simulink model "akku_schaetzung"  (R2021a)
settings: Solver=VariableStepAuto  StartTime=0.0  StopTime=time_est  RelTol=1e-3
values from neighbouring files (symbols this model uses):
  a = param    [temp.m]    (also in toolbox_ident.m = phi'*phi\phi'*u_oc)
  current = main_data{cur_ind}.Values    [check_output.m]    (also in init.m; init_2.m; init_3.m; power_energy.m)
  Delta = 8e-3    (= 0.008)    [check_output.m]    (also in init.m = volt_clean.Time(2)-volt_clean.Time(1); init_2.m; temp.m; toolbox_ident.m)
  P0 = eye(5); P0(1,1)=(0.03*x0(1))^2;P0(2,2)=(0.03*x0(2))^2;P0(3,3)=(0.03*x0(3))^2    [check_output.m]    (also in init.m; init_2.m; init_3.m = eye(6); P0(1,1)=(0.03*x0(1))^2;P0(2,2)=(0.03*x0(2))^2;P0(3,3; temp.m)
  Q_e = 2.9*3600    (= 10440)    [check_output.m]    (also in init_2.m; temp.m; toolbox_ident.m)
  voltage = main_data{volt_ind}.Values    [check_output.m]    (also in init.m; init_2.m; init_3.m; power_energy.m)
  W_k = 0.0*eye(5)    [check_output.m]    (also in init.m = 0.0*eye(6); init_2.m; init_3.m = 0.0*eye(6); temp.m)
  x0 = [1/param_conv(1); 1/param_conv(2); 1/param_conv(3); soc_0; 0]    [check_output.m]    (also in init.m = [1/790.27; 1/0.0126; 1/0.0086; 1/(2.9*3600); 0.5; 0]; init_2.m = [2/790.27; 1/0.0126/2; 1/0.0086/2; 0.5; 0]; init_3.m = [2/790.27; 1/2/0.0126; 1/2/0.0086; 1/(2.9*3600); 0.5; 0]; temp.m = [2/790.27; 1/0.0126/2; 1/0.0086/2; 0.5; 0])
  Z_k = var(static_volt)    [check_output.m]    (also in init.m = 0.02; init_2.m; init_3.m; temp.m)
undefined symbols (not defined in the file or in its folder): ind_val
libraries: simulink x2
settings Model: Creator=saleh  LastModifiedBy=saleh
settings SolverCC: AlgebraicLoopSolver=TrustRegion
settings DebuggingCC: SFMachineParentedDataDiag=warning

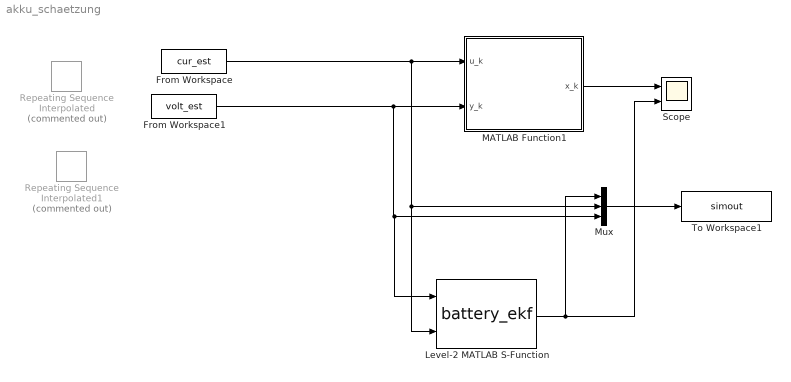
== system akku_schaetzung ==
  From Workspace : FromWorkspace  VariableName=cur_est  SampleTime=Delta
  From Workspace1 : FromWorkspace  VariableName=volt_est  SampleTime=Delta
  Level-2 MATLAB S-Function : M-S-Function  FunctionName=battery_ekf  Parameters=Delta, x0, P0, a, Z_k, W_k, Q_e
  MATLAB Function1 : MATLAB Function  TreatAsAtomicUnit=on
  Mux : Mux  Inputs=3
  Repeating Sequence Interpolated : simulink/Sources/Repeating Sequence Interpolated  Commented=on  OutValues=current.Data(1:ind_val)  TimeValues=current.Time(1:ind_val)  LookUpMeth=Interpolation-Use End Values  tsamp=Delta  OutMin=[]  OutMax=[]  OutDataTypeStr=double  OutputDataTypeScalingMode=double  OutDataType=fixdt(0,8)  OutScaling=2^-10
  Repeating Sequence Interpolated1 : simulink/Sources/Repeating Sequence Interpolated  Commented=on  OutValues=voltage.Data(1:ind_val)  TimeValues=voltage.Time(1:ind_val)  LookUpMeth=Interpolation-Use End Values  tsamp=Delta  OutMin=[]  OutMax=[]  OutDataTypeStr=double  OutputDataTypeScalingMode=double  OutDataType=fixdt(0,8)  OutScaling=2^-10
  Scope : Scope  NumInputPorts=2
  To Workspace1 : ToWorkspace  VariableName=simout  SampleTime=-1
  wires:
  From Workspace/1 -> Level-2 MATLAB S-Function/2, Mux/2, MATLAB Function1/1(u_k)
  From Workspace1/1 -> Level-2 MATLAB S-Function/1, Mux/3, MATLAB Function1/2(y_k)
  MATLAB Function1/1(x_k) -> Scope/1
  Mux/1 -> To Workspace1/1
  Level-2 MATLAB S-Function/1 -> Mux/1, Scope/2

== matlab function akku_schaetzung/MATLAB Function1 ==
  data: u_k input; x_k output; y_k input; x0 parameter; P0 parameter; W_k parameter; Z_k parameter; Delta parameter; a parameter; Q_e parameter
function x_k = ekf_2(u_k, y_k, x0, P0, W_k, Z_k, Delta, a, Q_e)
    
    persistent P_pk x_pk
    if isempty(x_pk)
        x_pk = x0; %x[k|k-1]
    end
    if isempty(P_pk)
        P_pk = P0;
    end
    
    eta = 1;
    
    a1 = a(1);a2 = a(2); a3 = a(3);
    
    % Kalman-Gain and real Covariance Matrix
    % States (1/C, 1/R, 1/R0, SOC, Uc)
    y_hat_k = a1*x_pk(4)^2+a2*x_pk(4)+a3+x_pk(5)+u_k/x_pk(3);
    C_k = [0, 0, -u_k/x_pk(3)^2, 2*a1*x_pk(4)+a2, 1];
    K_k = P_pk*C_k'/(Z_k + C_k*P_pk*C_k');
    x_k = x_pk + K_k*(y_k - y_hat_k);
    P_k = P_pk - K_k*C_k*P_pk;

    % Calculate A, prediction of x and P
    A_k = [[eye(4); zeros(1,4)], [Delta*(u_k-x_k(5)*x_k(3));0;...
        -Delta*x_k(1)*x_k(5);0;1-Delta*x_k(1)*x_k(3)]];
    x_pkp1 = [x_k(1);x_k(2);x_k(3);x_k(4)+Delta*u_k/Q_e;...
    x_k(5)-Delta*x_k(1)*(x_k(5)*x_k(2)-u_k)];
    
    P_pkp1 = A_k*P_k*A_k' + W_k;
    
    % Update persistent variable
    x_pk = x_pkp1;
    P_pk = P_pkp1;
end
